simulink model "Attitude_Control_Test"  (R2017b)
settings: Solver=VariableStepAuto  StartTime=0.0  StopTime=10.0  RelTol=1e-3
libraries: NLGCToolbox x5, simulink x2
settings Model: Creator=hoang  LastModifiedBy=hoang

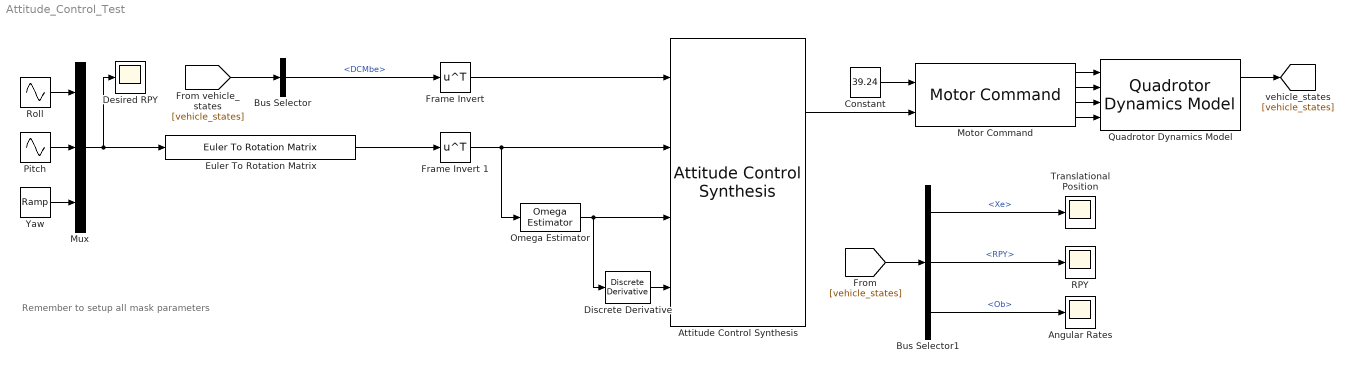
== system Attitude_Control_Test ==
  note: Remember to setup all mask parameters
  Angular Rates : Scope
  Attitude Control Synthesis : NLGCToolbox/Attitude Control Synthesis  quadrotor=quad  Ts1=1/120
      settings: SourceProductName=Thinh - NLGC for Quadrotor
  Bus Selector : BusSelector  OutputSignals=DCMbe
  Bus Selector1 : BusSelector  OutputSignals=Xe,RPY,Ob
  Constant : Constant  Value=39.24
  Desired RPY : Scope
  Discrete Derivative : simulink/Discrete/Discrete Derivative  gainval=1.0  ICPrevScaledInput=0.0  OutMin=[]  OutMax=[]  OutDataType=fixdt(1, 16)  OutScaling=2^-10  DoSatur=off
  Euler To Rotation Matrix : NLGCToolbox/Euler To Rotation Matrix
      settings: SourceProductName=Thinh - NLGC for Quadrotor
  Frame Invert : Math  Operator=transpose  SaturateOnIntegerOverflow=on
  Frame Invert 1 : Math  Operator=transpose  SaturateOnIntegerOverflow=on
  Motor Command : NLGCToolbox/Motor Command  quadrotor=quad
      settings: SourceProductName=Thinh - NLGC for Quadrotor
  Mux : Mux  Inputs=3
  Omega Estimator : NLGCToolbox/Omega Estimator  Ts=1/120
      settings: SourceProductName=Thinh - NLGC for Quadrotor
  Pitch : Sin  Amplitude=0.005  Frequency=2*pi/10  Phase=-pi/2  SampleTime=0
  Quadrotor Dynamics Model : NLGCToolbox/Quadrotor Dynamics Model  xinit=[0;0;-4]  quadrotor=quad
      settings: SourceProductName=Thinh - NLGC for Quadrotor
  RPY : Scope
  Roll : Sin  Amplitude=0.005  Frequency=2*pi/10  SampleTime=0
  Translational Position : Scope
  Yaw : simulink/Sources/Ramp  slope=0.05  start=0  X0=0
  wires:
  Motor Command/1 -> Quadrotor Dynamics Model/1
  Motor Command/2 -> Quadrotor Dynamics Model/2
  Motor Command/3 -> Quadrotor Dynamics Model/3
  Motor Command/4 -> Quadrotor Dynamics Model/4
  Attitude Control Synthesis/1 -> Motor Command/2
  Quadrotor Dynamics Model/1 -> [vehicle_states]
  [vehicle_states] -> Bus Selector/1
  Bus Selector/1 -> Frame Invert/1  "<DCMbe>"
  Frame Invert/1 -> Attitude Control Synthesis/1
  Euler To Rotation Matrix/1 -> Frame Invert 1/1
  Frame Invert 1/1 -> Omega Estimator/1, Attitude Control Synthesis/2
  Roll/1 -> Mux/1
  Pitch/1 -> Mux/2
  Yaw/1 -> Mux/3
  Mux/1 -> Desired RPY/1, Euler To Rotation Matrix/1
  Omega Estimator/1 -> Discrete Derivative/1, Attitude Control Synthesis/3
  Discrete Derivative/1 -> Attitude Control Synthesis/4
  Constant/1 -> Motor Command/1
  [vehicle_states] -> Bus Selector1/1
  Bus Selector1/2 -> RPY/1  "<RPY>"
  Bus Selector1/3 -> Angular Rates/1  "<Ob>"
  Bus Selector1/1 -> Translational Position/1  "<Xe>"
